simulink model "RackAndPinion"  (R2023a)
settings: Solver=VariableStepAuto  StartTime=0.0  StopTime=10.0  RelTol=1e-3
settings Model: Creator=Waffle  LastModifiedBy=Waffle

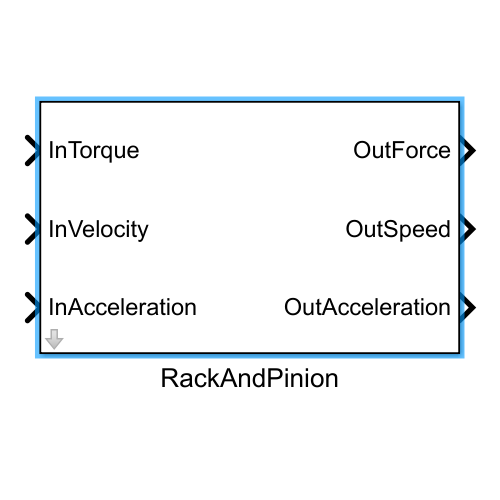
[thumbnail: Simulink's stored preview of the top-level diagram]
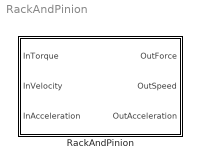
== system RackAndPinion ==
  RackAndPinion : Subsystem  mask{vis_friction_coef_gear=0.5, i_rack=20000, J_rack=0.000001, m=0.3}
      mask prompts: vis_friction_coef_gear "Коэф. вязкого трения"; i_rack "Передаточное отношение, рад/м"; J_rack "Момент инерции"; m "Масса маятника, кг"

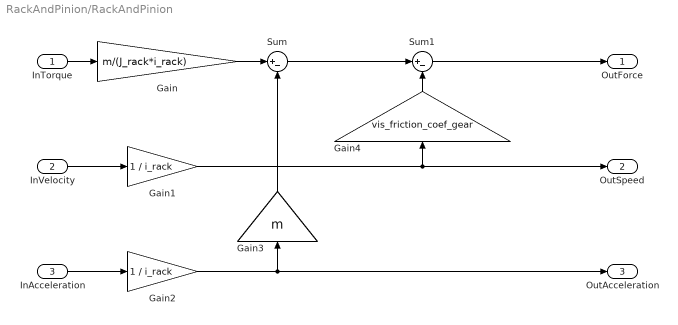
== system RackAndPinion/RackAndPinion ==
  InTorque : Inport
  InVelocity : Inport  Port=2
  InAcceleration : Inport  Port=3
  Gain : Gain  Gain=m/(J_rack*i_rack)
  Gain1 : Gain  Gain=1 / i_rack
  Gain2 : Gain  Gain=1 / i_rack
  Gain3 : Gain  Gain=m
  Gain4 : Gain  Gain=vis_friction_coef_gear
  Sum : Sum  Inputs=|+-
  Sum1 : Sum  Inputs=|+-
  OutForce : Outport
  OutSpeed : Outport  Port=2
  OutAcceleration : Outport  Port=3
  wires:
  InTorque/1 -> Gain/1
  InVelocity/1 -> Gain1/1
  InAcceleration/1 -> Gain2/1
  Gain2/1 -> Gain3/1, OutAcceleration/1
  Gain1/1 -> Gain4/1, OutSpeed/1
  Gain/1 -> Sum/1
  Sum/1 -> Sum1/1
  Sum1/1 -> OutForce/1
  Gain3/1 -> Sum/2
  Gain4/1 -> Sum1/2
